simulink model "wrench_observer"  (R2018b)
settings: Solver=VariableStepAuto  StartTime=0.0  StopTime=0.75  RelTol=1e-3
InitFcn:
  | %x_k1 = 0.00001*ones(36,1); % initialisation with initial state uncertainity
  | %P_k1 = 0.00001*ones(36); % initialisation with initial state uncertainity
values from neighbouring files (symbols this model uses):
  a_noise = 0    [parameter.m]
  alpha1 = pi/2    (= 1.57079632679)    [parameter.m]
  alpha2 = 0    [parameter.m]
  alpha3 = 0    [parameter.m]
  angular_noise = 0    [parameter.m]
  g = 9.81    [parameter.m]
  K_f_comm = 1    [parameter.m]
  K_I = [500*eye(3), zeros(3), zeros(3) ... (first row only)    [parameter.m]
  K_tau_comm = 1    [parameter.m]
  K_tau_man_comm = 1    [parameter.m]
  m = 3.9    [parameter.m]
  m_l1 = 0.3    [parameter.m]
  m_l2 = 0.35    [parameter.m]
  m_l3 = 0.35    [parameter.m]
  N_m = 1*diag([(p_noise/(3*noise_factor))^2 (p_noise/(3*noise_factor))^2 (p_noise/(3*noise_factor))^2 (a_noise/(3*noise_factor))^2 (a_noise/(3*noise_factor))^2 (a_noise/(3*noise_factor))^2 (angular_noise/(3*noise_factor))^2 (angular_noise/(3*noise_factor))^2 (angular_noise/(3*noise_factor))^2 (omega_noise/(3*noise_factor))^2 (omega_noise/(3*noise_factor))^2 (omega_noise/(3*noise_factor))^2 (theta_noise/( ...(+272 chars)    [parameter.m]
  N_p = diag(noise_factor_EKF)    [parameter.m]
  omega_dot_noise = 0    [parameter.m]
  omega_noise = 0    [parameter.m]
  p_L1_l1 = [p_L1_x_l1 p_L1_y_l1 p_L1_z_l1]'    [parameter.m]
  p_L2_l2 = [p_L2_x_l2 p_L2_y_l2 p_L2_z_l2]'    [parameter.m]
  p_L3_l3 = [p_L3_x_l3 p_L3_y_l3 p_L3_z_l3]'    [parameter.m]
  p_noise = 0    [parameter.m]
  R_B_L0 = [1 0 0;0 1 0; 0 0 1]    [parameter.m]
  T_delay = 0    [parameter.m]
  T_dis = 0.01    [parameter.m]
  theta_dot_dot_noise = 0    [parameter.m]
  theta_dot_noise = 0    [parameter.m]
  theta_noise = 0    [parameter.m]
  Ts = 1/250    (= 0.004)    [parameter.m]
  v_noise = 0    [parameter.m]
libraries: simulink x9, dspstat3 x2, dspinverses x1
(part 5 of 5)

== matlab function wrench_observer/Motion Equations with Manipulator /MATLAB Function2 ==
  data: q input; G output; alpha1 parameter; alpha2 parameter; alpha3 parameter; R_B_L0 parameter; g parameter; m parameter; m_l2 parameter; m_l3 parameter; m_l1 parameter; p_L1_l1 parameter; p_L2_l2 parameter; p_L3_l3 parameter
function G = Gravity_Matrix(q, alpha1, alpha2, alpha3, R_B_L0, g, m, m_l2, m_l3, m_l1, p_L1_l1, p_L2_l2, p_L3_l3)
phi_E = q(4);
theta_E = q(5);
psi_E = q(6);
theta1 = q(7);
theta2 = q(8);
theta3 = q(9);
% theta4 = q(10);
% theta5 = q(11);

sphi = sin(phi_E); cphi = cos(phi_E);
sth = sin(theta_E); cth = cos(theta_E);
spsi = sin(psi_E); cpsi = cos(psi_E);
sth1 = sin(theta1); cth1 = cos(theta1); sth2 = sin(theta2); cth2 = cos(theta2); sth3 = sin(theta3); cth3 = cos(theta3);
salp1 = sin(alpha1); calp1 = cos(alpha1); salp2 = sin(alpha2); calp2 = cos(alpha2); salp3 = sin(alpha3); calp3 = cos(alpha3);

p_L1_x_l1 = p_L1_l1(1); p_L1_y_l1 = p_L1_l1(2); p_L1_z_l1 = p_L1_l1(3);
p_L2_x_l2 = p_L2_l2(1); p_L2_y_l2 = p_L2_l2(2); p_L2_z_l2 = p_L2_l2(3);
p_L3_x_l3 = p_L3_l3(1); p_L3_y_l3 = p_L3_l3(2); p_L3_z_l3 = p_L3_l3(3);
%% Rotation matrix from inertial to body frame
R_IB = [cpsi*cth cpsi*sth*sphi-spsi*cphi cpsi*sth*cphi+spsi*sphi;
        spsi*cth spsi*sth*sphi+cpsi*cphi spsi*sth*cphi-cpsi*sphi;
        -sth cth*sphi cth*cphi];

%% Rotation matrices from link i to manipulator base {L0}
% R_th_1 = [cth1 -sth1 0 0;
%     sth1 cth1 0 0;
%     0 0 1 0;
%     0 0 0 1];
% R_alpha_1 = [1 0 0 0;
%     0 calp1 -salp1 0;
%     0 salp1 calp1 0;
%     0 0 0 1];
% R_th_2 = [cth2 -sth2 0 0;
%     sth2 cth2 0 0;
%     0 0 1 0;
%     0 0 0 1];
% R_alpha_2 = [1 0 0 0;
%     0 calp2 -salp2 0;
%     0 salp2 calp2 0;
%     0 0 0 1];
% R_th_3 = [cth3 -sth3 0 0;
%     sth3 cth3 0 0;
%     0 0 1 0;
%     0 0 0 1];
% R_alpha_3 = [1 0 0 0;
%     0 calp3 -salp3 0;
%     0 salp3 calp3 0;
%     0 0 0 1];
% R_th_4 = [cth4 -sth4 0 0;
%         sth4 cth4 0 0;
%         0 0 1 0;
%         0 0 0 1];
% R_alpha_4 = [1 0 0 0;
%            0 calph4 -salph4 0;
%            0 salph4 calph4 0;
%            0 0 0 1];
% R_th_5 = [cth5 -sth5 0 0;
%         sth5 cth5 0 0;
%         0 0 1 0;
%         0 0 0 1];
% R_alpha_5 = [1 0 0 0;
%            0 calph5 -salph5 0;
%            0 salph5 calph5 0;
%            0 0 0 1];

% transformation matrices from link i to link i-1
% T_L0_L1 = R_th_1 * [1 0 0 0;0 1 0 0;0 0 1 d1;0 0 0 0] * [1 0 0 a1;0 1 0 0;0 0 1 0;0 0 0 1] * R_alpha_1;
% T_L1_L2 = R_th_2 * [1 0 0 0;0 1 0 0;0 0 1 d2;0 0 0 0] * [1 0 0 a2;0 1 0 0;0 0 1 0;0 0 0 1] * R_alpha_2;
% T_L2_L3 = R_th_3 * [1 0 0 0;0 1 0 0;0 0 1 d3;0 0 0 0] * [1 0 0 a3;0 1 0 0;0 0 1 0;0 0 0 1] * R_alpha_3;
% T_L3_L4 = R_th_4 * [1 0 0 0;0 1 0 0;0 0 1 d4;0 0 0 0] * [1 0 0 a4;0 1 0 0;0 0 1 0;0 0 0 1] * R_alpha_4;
% T_L4_L5 = R_th_5 * [1 0 0 0;0 1 0 0;0 0 1 d5;0 0 0 0] * [1 0 0 a5;0 1 0 0;0 0 1 0;0 0 0 1] * R_alpha_5;

% transformatin matrices from link i to manipulator base {L0}
% T_L0_L2 = T_L0_L1*T_L1_L2;
% T_L0_L3 = T_L0_L2*T_L2_L3;
% T_L0_L4 = T_L0_L3*T_L3_L4;
% T_L0_L5 = T_L0_L4*T_L4_L5;

% rotation matrices from link i to manipulator base {L0}
% R_L0_L1 = T_L0_L1(1:3,1:3);
% R_L0_L2 = T_L0_L2(1:3,1:3);
% R_L0_L3 = T_L0_L3(1:3,1:3);
% R_L0_L4 = T_L0_L4(1:3,1:3);
% R_L0_L5 = T_L0_L5(1:3,1:3);

R_L0_L1 = [ cth1, -calp1*sth1,  sth1*salp1;
            sth1,  cth1*calp1, -cth1*salp1;
             0,         salp1,       calp1];

R_L0_L2 = [ cth1*cth2 - calp1*sth1*sth2, sth1*salp1*salp2 - cth1*calp2*sth2 - cth2*calp1*calp2*sth1, cth1*sth2*salp2 + calp2*sth1*salp1 + cth2*calp1*sth1*salp2;
            cth2*sth1 + cth1*calp1*sth2, cth1*cth2*calp1*calp2 - cth1*salp1*salp2 - calp2*sth1*sth2, sth1*sth2*salp2 - cth1*calp2*salp1 - cth1*cth2*calp1*salp2;
             sth2*salp1,                                                   calp1*salp2 + cth2*calp2*salp1,                       calp1*calp2 - cth2*salp1*salp2];
         
R_L0_L3 = [ cth3*(cth1*cth2 - calp1*sth1*sth2) - sth3*(calp2*cth1*sth2 - salp1*salp2*sth1 + calp1*calp2*cth2*sth1),   salp3*(calp2*salp1*sth1 + salp2*cth1*sth2 + calp1*salp2*cth2*sth1) - calp3*cth3*(calp2*cth1*sth2 - salp1*salp2*sth1 + calp1*calp2*cth2*sth1) - calp3*sth3*(cth1*cth2 - calp1*sth1*sth2), calp3*(calp2*salp1*sth1 + salp2*cth1*sth2 + calp1*salp2*cth2*sth1) + salp3*cth3*(calp2*cth1*sth2 - salp1*salp2*sth1 + calp1*calp2*cth2*sth1) + salp3*sth3*(cth1*cth2 - calp1*sth1*sth2);
            cth3*(cth2*sth1 + calp1*cth1*sth2) - sth3*(salp1*salp2*cth1 + calp2*sth1*sth2 - calp1*calp2*cth1*cth2), - salp3*(calp2*salp1*cth1 - salp2*sth1*sth2 + calp1*salp2*cth1*cth2) - calp3*cth3*(salp1*salp2*cth1 + calp2*sth1*sth2 - calp1*calp2*cth1*cth2) - calp3*sth3*(cth2*sth1 + calp1*cth1*sth2), salp3*cth3*(salp1*salp2*cth1 + calp2*sth1*sth2 - calp1*calp2*cth1*cth2) - calp3*(calp2*salp1*cth1 - salp2*sth1*sth2 + calp1*salp2*cth1*cth2) + salp3*sth3*(cth2*sth1 + calp1*cth1*sth2);
             sth3*(calp1*salp2 + calp2*salp1*cth2) + salp1*cth3*sth2,                                                                                                                                      salp3*(calp1*calp2 - salp1*salp2*cth2) + calp3*cth3*(calp1*salp2 + calp2*salp1*cth2) - calp3*salp1*sth2*sth3,                                                                 calp3*(calp1*calp2 - salp1*salp2*cth2) - salp3*cth3*(calp1*salp2 + calp2*salp1*cth2) + salp1*salp3*sth2*sth3];

%% Gravity vector
a = R_B_L0(1,1)*R_IB(3,1)+ R_B_L0(2,1)*R_IB(3,2)+ R_B_L0(3,1)*R_IB(3,3);
b = R_B_L0(1,2)*R_IB(3,1)+ R_B_L0(2,2)*R_IB(3,2)+ R_B_L0(3,2)*R_IB(3,3);
c = R_B_L0(1,3)*R_IB(3,1)+ R_B_L0(2,3)*R_IB(3,2)+ R_B_L0(3,3)*R_IB(3,3);
% partial derivatives
dadphi = -R_B_L0(2,1)*cphi*cth + R_B_L0(3,1)*sphi*cth;
dadth = R_B_L0(1,1)*cth + R_B_L0(2,1)*sphi*sth + R_B_L0(3,1)*cphi*sth;
dadpsi = 0;
dbdphi = -R_B_L0(2,2)*cphi*cth + R_B_L0(3,2)*sphi*cth;
dbdth = R_B_L0(1,2)*cth + R_B_L0(2,2)*sphi*sth + R_B_L0(3,2)*cphi*sth;
dbdpsi = 0;
dcdphi = -R_B_L0(2,3)*cphi*cth + R_B_L0(3,3)*sphi*cth;
dcdth = R_B_L0(1,3)*cth + R_B_L0(2,3)*sphi*sth + R_B_L0(3,3)*cphi*sth;
dcdpsi = 0;

% gravity vector UAV
dUuav = [0 0 g*m 0 0 0 0 0 0]';
% gravity vector link 1
dUman_1 = zeros(9,1);
dUman_1(1) = 0; dUman_1(2) = 0; dUman_1(3) = g*m_l1;
dUman_1(4) = p_L1_x_l1*m_l1*g*(R_L0_L1(1,1)*dadphi + R_L0_L1(2,1)*dbdphi + R_L0_L1(3,1)*dcdphi)                                       + p_L1_y_l1*m_l1*g*(R_L0_L1(1,2)*dadphi + R_L0_L1(2,2)*dbdphi + R_L0_L1(3,2)*dcdphi)      + p_L1_z_l1*m_l1*g*(R_L0_L1(1,3)*dadphi + R_L0_L1(2,3)*dbdphi + R_L0_L1(3,3)*dcdphi);
dUman_1(5) = p_L1_x_l1*m_l1*g*(R_L0_L1(1,1)*dadth + R_L0_L1(2,1)*dbdth + R_L0_L1(3,1)*dcdth)                                          + p_L1_y_l1*m_l1*g*(R_L0_L1(1,2)*dadth + R_L0_L1(2,2)*dbdth + R_L0_L1(3,2)*dcdth)         + p_L1_z_l1*m_l1*g*(R_L0_L1(1,3)*dadth + R_L0_L1(2,3)*dbdth + R_L0_L1(3,3)*dcdth);
dUman_1(6) = p_L1_x_l1*m_l1*g*(R_L0_L1(1,1)*dadpsi + R_L0_L1(2,1)*dbdpsi + R_L0_L1(3,1)*dcdpsi)                                       + p_L1_y_l1*m_l1*g*(R_L0_L1(1,2)*dadpsi + R_L0_L1(2,2)*dbdpsi + R_L0_L1(3,2)*dcdpsi)      + p_L1_z_l1*m_l1*g*(R_L0_L1(1,3)*dadpsi + R_L0_L1(2,3)*dbdpsi + R_L0_L1(3,3)*dcdpsi);
dUman_1(7) = p_L1_x_l1*m_l1*g*(sth1*a - cth1*b)                                                                                       + p_L1_y_l1*m_l1*g*(-cth1*calp1*a + sth1*calp1*b)                                         + p_L1_z_l1*m_l1*g*(cth1*salp1*a + sth1*salp1*b);
dUman_1(8) = 0;
dUman_1(9) = 0;
% gravity vector link 2
dUman_2 = zeros(9,1);
dUman_2(1) = 0; dUman_2(2) = 0; dUman_2(3) = g*m_l2;
dUman_2(4) = p_L2_x_l2*m_l2*g*(R_L0_L2(1,1)*dadphi + R_L0_L2(2,1)*dbdphi + R_L0_L2(3,1)*dcdphi)                                       + p_L2_y_l2*m_l2*g*(R_L0_L2(1,2)*dadphi + R_L0_L2(2,2)*dbdphi + R_L0_L2(3,2)*dcdphi)                                                                  + p_L2_z_l2*m_l2*g*(R_L0_L2(1,3)*dadphi + R_L0_L2(2,3)*dbdphi + R_L0_L2(3,3)*dcdphi);
dUman_2(5) = p_L2_x_l2*m_l2*g*(R_L0_L2(1,1)*dadth + R_L0_L2(2,1)*dbdth + R_L0_L2(3,1)*dcdth)                                          + p_L2_y_l2*m_l2*g*(R_L0_L2(1,2)*dadth + R_L0_L2(2,2)*dbdth + R_L0_L2(3,2)*dcdth)                                                                     + p_L2_z_l2*m_l2*g*(R_L0_L2(1,3)*dadth + R_L0_L2(2,3)*dbdth + R_L0_L2(3,3)*dcdth);
dUman_2(6) = p_L2_x_l2*m_l2*g*(R_L0_L2(1,1)*dadpsi + R_L0_L2(2,1)*dbdpsi + R_L0_L2(3,1)*dcdpsi)                                       + p_L2_y_l2*m_l2*g*(R_L0_L2(1,2)*dadpsi + R_L0_L2(2,2)*dbdpsi + R_L0_L2(3,2)*dcdpsi)                                                                  + p_L2_z_l2*m_l2*g*(R_L0_L2(1,3)*dadpsi + R_L0_L2(2,3)*dbdpsi + R_L0_L2(3,3)*dcdpsi);
dUman_2(7) = p_L2_x_l2*m_l2*g*((sth1*cth2+cth1*sth2*calp1)*a + (-cth1*cth2+sth1*sth2*calp1)*b)                                        + p_L2_y_l2*m_l2*g*((-cth1*salp1*salp2-sth1*sth2*calp2+cth1*cth2*calp1*calp2)*a + (sth1*cth2*calp1*calp2-sth1*salp1*salp2+cth1*sth2*calp2)*b)         + p_L2_z_l2*m_l2*g*((sth1*sth2*salp2-cth2*salp1*calp2-cth1*cth2*calp1*salp2)*a + (-cth1*sth2*salp2-sth1*salp1*calp2-sth1*cth2*calp1*salp2)*b);
dUman_2(8) = p_L2_x_l2*m_l2*g*((sth2*cth1+cth2*sth1*calp1)*a + (sth2*sth1-cth2*cth1*calp1)*b + (-cth2*salp1)*c)                       + p_L2_y_l2*m_l2*g*((cth2*cth1*calp2-sth2*sth1*calp1*calp2)*a + (sth2*cth1*calp1*calp2+cth2*sth1*calp2)*b + (sth2*salp1*calp2)*c)                     + p_L2_z_l2*m_l2*g*((-cth2*cth1*salp2+sth2*sth1*calp1*salp2)*a + (-cth2*sth1*salp2)*b + (-sth2*salp1*salp2)*c);
dUman_2(9) = 0;
% gravity vector link 3
dUman_3 = zeros(9,1);
dUman_3(1) = 0; dUman_3(2) = 0; dUman_3(3) = g*m_l3;
dUman_3(4) = p_L3_x_l3*m_l3*g*(R_L0_L3(1,1)*dadphi + R_L0_L3(2,1)*dbdphi + R_L0_L3(3,1)*dcdphi)                                                                                                                                                                                                         + p_L3_y_l3*m_l3*g*(R_L0_L3(1,2)*dadphi + R_L0_L3(2,2)*dbdphi + R_L0_L3(3,2)*dcdphi)                                                                                                                                                                                                                                                                                            + p_L3_z_l3*m_l3*g*(R_L0_L3(1,3)*dadphi + R_L0_L3(2,3)*dbdphi + R_L0_L3(3,3)*dcdphi);
dUman_3(5) = p_L3_x_l3*m_l3*g*(R_L0_L3(1,1)*dadth + R_L0_L3(2,1)*dbdth + R_L0_L3(3,1)*dcdth)                                                                                                                                                                                                            + p_L3_y_l3*m_l3*g*(R_L0_L3(1,2)*dadth + R_L0_L3(2,2)*dbdth + R_L0_L3(3,2)*dcdth)                                                                                                                                                                                                                                                                                               + p_L3_z_l3*m_l3*g*(R_L0_L3(1,3)*dadth + R_L0_L3(2,3)*dbdth + R_L0_L3(3,3)*dcdth);
dUman_3(6) = p_L3_x_l3*m_l3*g*(R_L0_L3(1,1)*dadpsi + R_L0_L3(2,1)*dbdpsi + R_L0_L3(3,1)*dcdpsi)                                                                                                                                                                                                         + p_L3_y_l3*m_l3*g*(R_L0_L3(1,2)*dadpsi + R_L0_L3(2,2)*dbdpsi + R_L0_L3(3,2)*dcdpsi)                                                                                                                                                                                                                                                                                            + p_L3_z_l3*m_l3*g*(R_L0_L3(1,3)*dadpsi + R_L0_L3(2,3)*dbdpsi + R_L0_L3(3,3)*dcdpsi);
dUman_3(7) = p_L3_x_l3*m_l3*g*((sth1*cth2*cth3+cth1*sth2*calp1-sth1*sth2*sth3*calp2+cth1*salp1*salp2-cth1*cth2*calp1*calp2)*a + (cth1*cth2*cth3+cth1*sth2*calp1+cth1*sth2*sth3*calp2-sth1*salp1*salp2-sth1*cth2*calp1*calp2)*b)                                                                         + p_L3_y_l3*m_l3*g*((sth1*sth2*salp2*salp3-cth1*salp1*calp2-cth1*cth2*calp1*calp2-sth1*sth2*cth3*calp2*calp3+cth1*salp1*salp2-cth1*cth2*calp1*calp2-sth1*cth2*sth3*calp3+cth1*sth2*calp1)*a + (-sth1*salp1*calp2*salp3+cth1*sth2*salp2+sth1*cth2*calp1*salp2+cth1*sth2*cth3*calp2*calp3+sth1*salp1*salp2-sth1*cth2*calp1*calp2+cth1*cth2*sth3*calp3+sth1*sth2*calp1)*b)         + p_L3_z_l3*m_l3*g*((sth1*sth2*salp2*calp3-cth1*salp1*calp2-cth1*cth2*calp1*salp2+sth1*sth2*cth3*calp2*salp3+cth1*salp1*salp2-cth1*cth2*calp1*calp2+sth1*cth2*sth3*salp3+cth1*sth2*calp1)*a + (-cth1*sth2*cth3*calp2*salp3+sth1*salp1*salp2-sth1*cth2*calp1*calp2-sth1*salp1*calp2*calp3+cth1*sth2*salp2+sth1*cth2*calp1*salp2-cth1*cth2*sth3*salp3+sth1*sth2*calp1)*b);
dUman_3(8) = p_L3_x_l3*m_l3*g*((sth2*cth1*cth3+cth2*sth1*calp1+cth2*cth1*sth3*calp2+sth2*sth1*calp1)*a + (sth2*sth1*cth3-cth2*cth1*calp1+cth2*sth1*sth3*calp2-sth2*cth1*calp1*calp2)*b + (-cth2*cth3*salp1+sth2*sth3*salp1*calp2)*c)                                                                    + p_L3_y_l3*m_l3*g*((-cth2*cth1*salp2*salp3+sth2*sth1*calp1-sth2*cth1*sth3*calp3+cth2*sth1*calp1+cth2*cth1*cth3*calp2*calp3+sth2*sth1*calp1)*a + (-cth2*sth1*salp2*salp3-sth2*cth1*calp1-sth2*sth1*sth3*calp3-cth2*cth1*calp1+cth2*sth1*cth3*calp2*calp3-sth2*cth1*calp1)*b + (sth2*cth3*salp1*calp2*calp3+cth2*sth3*salp1*calp3-sth2*salp1*salp2*salp3)*c)                     + p_L3_z_l3*m_l3*g*((sth2*cth1*sth3*salp3+cth2*sth1*calp1-cth2*cth1*salp2*calp3+sth2*sth1*calp1-cth2*cth1*cth3*calp2*salp3+sth2*sth1*calp1)*a - (sth2*sth1*sth3*salp3-cth2*cth1*calp1-cth2*sth1*salp2*calp3-sth2*cth1*calp1-cth2*sth1*cth3*calp2*salp3-sth2*cth1*calp1)*b + (-cth2*sth3*salp1*salp3-sth2*salp1*salp2*calp3-sth2*cth3*salp1*calp2*salp3)*c);
dUman_3(9) = p_L3_x_l3*m_l3*g*((sth3*(cth1*cth2-sth1*sth2*calp1)+cth3*(cth1*sth2*calp2-sth1*salp1*salp2+sth1*cth2*calp1*calp2))*a + (sth3*(sth1*cth2+cth1*sth2*calp1)+cth3*(cth1*salp1*salp2+sth1*sth2*calp2-cth1*cth2*calp1*calp2))*b + (-cth3*(calp1*salp2+cth2*salp1*calp2)+sth3*sth2*salp1)*c)      + p_L3_y_l3*m_l3*g*((-sth3*calp3*(cth1*sth2*calp2-sth1*salp1*salp2+sth1*cth2*calp1*calp2-calp3*(cth1*cth2-sth1*sth2*calp1))*a + (-sth3*calp3*(cth1*salp1*salp2+sth1*sth2*calp2-cth1*cth2*calp1*calp2+cth3*calp3*(sth1*cth2+cth1*sth2*calp1)))*b + (-sth3*calp3*(calp1*salp2+cth2*salp1*calp2)+cth3*sth2*salp1*calp3))*c)                                                        + p_L3_z_l3*m_l3*g*((sth3*salp3*(cth1*sth2*calp2-sth1*salp1*salp2+sth1*cth2*calp1*calp2)-cth3*salp3*(cth1*cth2-sth1*sth2*calp1)))*a +(sth3*salp3*(cth1*salp1*salp2+sth1*sth2*calp2-cth1*cth2+calp1*calp2)-cth3*salp3*(sth1*cth2+cth1*sth2*calp1))*b + (-cth3*sth2*salp1*salp3-sth3*salp3*(calp1*salp2+cth2*salp1*calp2)*c);

G = dUuav + dUman_1 + dUman_2 + dUman_3;

== matlab function wrench_observer/Wrench Observer Hybrid Observer/Coriolis_Matrix/Coriolis_Matrix_simplified/MATLAB Function ==
  data: C11 input; C output; C12 input; C13 input; C21 input; C22 input; C23 input; C31 input; C32 input; C33 input
function C = Coriolis_Matrix(C11,C12,C13,C21,C22,C23,C31,C32,C33)
C = zeros(9);
C = [C11,C12,C13;C21,C22,C23;C31,C32,C33];

== matlab function wrench_observer/Wrench Observer Hybrid Observer/MATLAB Function2 ==
  data: q_meas input; G_est output; alpha1 parameter; alpha2 parameter; alpha3 parameter; R_B_L0 parameter; g parameter; m parameter; m_l2 parameter; m_l3 parameter; m_l1 parameter; p_L1_l1 parameter; p_L2_l2 parameter; p_L3_l3 parameter
function G_est = Gravity_Matrix(q_meas, alpha1, alpha2, alpha3, R_B_L0, g, m, m_l2, m_l3, m_l1, p_L1_l1, p_L2_l2, p_L3_l3)
phi_E = q_meas(4);
theta_E = q_meas(5);
psi_E = q_meas(6);
theta1 = q_meas(7);
theta2 = q_meas(8);
theta3 = q_meas(9);
% theta4 = q(10);
% theta5 = q(11);

sphi = sin(phi_E); cphi = cos(phi_E);
sth = sin(theta_E); cth = cos(theta_E);
spsi = sin(psi_E); cpsi = cos(psi_E);
sth1 = sin(theta1); cth1 = cos(theta1); sth2 = sin(theta2); cth2 = cos(theta2); sth3 = sin(theta3); cth3 = cos(theta3);
salp1 = sin(alpha1); calp1 = cos(alpha1); salp2 = sin(alpha2); calp2 = cos(alpha2); salp3 = sin(alpha3); calp3 = cos(alpha3);

p_L1_x_l1 = p_L1_l1(1); p_L1_y_l1 = p_L1_l1(2); p_L1_z_l1 = p_L1_l1(3);
p_L2_x_l2 = p_L2_l2(1); p_L2_y_l2 = p_L2_l2(2); p_L2_z_l2 = p_L2_l2(3);
p_L3_x_l3 = p_L3_l3(1); p_L3_y_l3 = p_L3_l3(2); p_L3_z_l3 = p_L3_l3(3);
%% Rotation matrix from inertial to body frame
R_IB = [cpsi*cth cpsi*sth*sphi-spsi*cphi cpsi*sth*cphi+spsi*sphi;
        spsi*cth spsi*sth*sphi+cpsi*cphi spsi*sth*cphi-cpsi*sphi;
        -sth cth*sphi cth*cphi];

%% Rotation matrices from link i to manipulator base {L0}
% R_th_1 = [cth1 -sth1 0 0;
%     sth1 cth1 0 0;
%     0 0 1 0;
%     0 0 0 1];
% R_alpha_1 = [1 0 0 0;
%     0 calp1 -salp1 0;
%     0 salp1 calp1 0;
%     0 0 0 1];
% R_th_2 = [cth2 -sth2 0 0;
%     sth2 cth2 0 0;
%     0 0 1 0;
%     0 0 0 1];
% R_alpha_2 = [1 0 0 0;
%     0 calp2 -salp2 0;
%     0 salp2 calp2 0;
%     0 0 0 1];
% R_th_3 = [cth3 -sth3 0 0;
%     sth3 cth3 0 0;
%     0 0 1 0;
%     0 0 0 1];
% R_alpha_3 = [1 0 0 0;
%     0 calp3 -salp3 0;
%     0 salp3 calp3 0;
%     0 0 0 1];
% R_th_4 = [cth4 -sth4 0 0;
%         sth4 cth4 0 0;
%         0 0 1 0;
%         0 0 0 1];
% R_alpha_4 = [1 0 0 0;
%            0 calph4 -salph4 0;
%            0 salph4 calph4 0;
%            0 0 0 1];
% R_th_5 = [cth5 -sth5 0 0;
%         sth5 cth5 0 0;
%         0 0 1 0;
%         0 0 0 1];
% R_alpha_5 = [1 0 0 0;
%            0 calph5 -salph5 0;
%            0 salph5 calph5 0;
%            0 0 0 1];

% transformation matrices from link i to link i-1
% T_L0_L1 = R_th_1 * [1 0 0 0;0 1 0 0;0 0 1 d1;0 0 0 0] * [1 0 0 a1;0 1 0 0;0 0 1 0;0 0 0 1] * R_alpha_1;
% T_L1_L2 = R_th_2 * [1 0 0 0;0 1 0 0;0 0 1 d2;0 0 0 0] * [1 0 0 a2;0 1 0 0;0 0 1 0;0 0 0 1] * R_alpha_2;
% T_L2_L3 = R_th_3 * [1 0 0 0;0 1 0 0;0 0 1 d3;0 0 0 0] * [1 0 0 a3;0 1 0 0;0 0 1 0;0 0 0 1] * R_alpha_3;
% T_L3_L4 = R_th_4 * [1 0 0 0;0 1 0 0;0 0 1 d4;0 0 0 0] * [1 0 0 a4;0 1 0 0;0 0 1 0;0 0 0 1] * R_alpha_4;
% T_L4_L5 = R_th_5 * [1 0 0 0;0 1 0 0;0 0 1 d5;0 0 0 0] * [1 0 0 a5;0 1 0 0;0 0 1 0;0 0 0 1] * R_alpha_5;

% transformatin matrices from link i to manipulator base {L0}
% T_L0_L2 = T_L0_L1*T_L1_L2;
% T_L0_L3 = T_L0_L2*T_L2_L3;
% T_L0_L4 = T_L0_L3*T_L3_L4;
% T_L0_L5 = T_L0_L4*T_L4_L5;

% rotation matrices from link i to manipulator base {L0}
% R_L0_L1 = T_L0_L1(1:3,1:3);
% R_L0_L2 = T_L0_L2(1:3,1:3);
% R_L0_L3 = T_L0_L3(1:3,1:3);
% R_L0_L4 = T_L0_L4(1:3,1:3);
% R_L0_L5 = T_L0_L5(1:3,1:3);

R_L0_L1 = [ cth1, -calp1*sth1,  sth1*salp1;
            sth1,  cth1*calp1, -cth1*salp1;
             0,         salp1,       calp1];

R_L0_L2 = [ cth1*cth2 - calp1*sth1*sth2, sth1*salp1*salp2 - cth1*calp2*sth2 - cth2*calp1*calp2*sth1, cth1*sth2*salp2 + calp2*sth1*salp1 + cth2*calp1*sth1*salp2;
            cth2*sth1 + cth1*calp1*sth2, cth1*cth2*calp1*calp2 - cth1*salp1*salp2 - calp2*sth1*sth2, sth1*sth2*salp2 - cth1*calp2*salp1 - cth1*cth2*calp1*salp2;
             sth2*salp1,                                                   calp1*salp2 + cth2*calp2*salp1,                       calp1*calp2 - cth2*salp1*salp2];
         
R_L0_L3 = [ cth3*(cth1*cth2 - calp1*sth1*sth2) - sth3*(calp2*cth1*sth2 - salp1*salp2*sth1 + calp1*calp2*cth2*sth1),   salp3*(calp2*salp1*sth1 + salp2*cth1*sth2 + calp1*salp2*cth2*sth1) - calp3*cth3*(calp2*cth1*sth2 - salp1*salp2*sth1 + calp1*calp2*cth2*sth1) - calp3*sth3*(cth1*cth2 - calp1*sth1*sth2), calp3*(calp2*salp1*sth1 + salp2*cth1*sth2 + calp1*salp2*cth2*sth1) + salp3*cth3*(calp2*cth1*sth2 - salp1*salp2*sth1 + calp1*calp2*cth2*sth1) + salp3*sth3*(cth1*cth2 - calp1*sth1*sth2);
            cth3*(cth2*sth1 + calp1*cth1*sth2) - sth3*(salp1*salp2*cth1 + calp2*sth1*sth2 - calp1*calp2*cth1*cth2), - salp3*(calp2*salp1*cth1 - salp2*sth1*sth2 + calp1*salp2*cth1*cth2) - calp3*cth3*(salp1*salp2*cth1 + calp2*sth1*sth2 - calp1*calp2*cth1*cth2) - calp3*sth3*(cth2*sth1 + calp1*cth1*sth2), salp3*cth3*(salp1*salp2*cth1 + calp2*sth1*sth2 - calp1*calp2*cth1*cth2) - calp3*(calp2*salp1*cth1 - salp2*sth1*sth2 + calp1*salp2*cth1*cth2) + salp3*sth3*(cth2*sth1 + calp1*cth1*sth2);
             sth3*(calp1*salp2 + calp2*salp1*cth2) + salp1*cth3*sth2,                                                                                                                                      salp3*(calp1*calp2 - salp1*salp2*cth2) + calp3*cth3*(calp1*salp2 + calp2*salp1*cth2) - calp3*salp1*sth2*sth3,                                                                 calp3*(calp1*calp2 - salp1*salp2*cth2) - salp3*cth3*(calp1*salp2 + calp2*salp1*cth2) + salp1*salp3*sth2*sth3];

%% Gravity vector
a = R_B_L0(1,1)*R_IB(3,1)+ R_B_L0(2,1)*R_IB(3,2)+ R_B_L0(3,1)*R_IB(3,3);
b = R_B_L0(1,2)*R_IB(3,1)+ R_B_L0(2,2)*R_IB(3,2)+ R_B_L0(3,2)*R_IB(3,3);
c = R_B_L0(1,3)*R_IB(3,1)+ R_B_L0(2,3)*R_IB(3,2)+ R_B_L0(3,3)*R_IB(3,3);
% partial derivatives
dadphi = -R_B_L0(2,1)*cphi*cth + R_B_L0(3,1)*sphi*cth;
dadth = R_B_L0(1,1)*cth + R_B_L0(2,1)*sphi*sth + R_B_L0(3,1)*cphi*sth;
dadpsi = 0;
dbdphi = -R_B_L0(2,2)*cphi*cth + R_B_L0(3,2)*sphi*cth;
dbdth = R_B_L0(1,2)*cth + R_B_L0(2,2)*sphi*sth + R_B_L0(3,2)*cphi*sth;
dbdpsi = 0;
dcdphi = -R_B_L0(2,3)*cphi*cth + R_B_L0(3,3)*sphi*cth;
dcdth = R_B_L0(1,3)*cth + R_B_L0(2,3)*sphi*sth + R_B_L0(3,3)*cphi*sth;
dcdpsi = 0;

% gravity vector UAV
dUuav = [0 0 g*m 0 0 0 0 0 0]';
% gravity vector link 1
dUman_1 = zeros(9,1);
dUman_1(1) = 0; dUman_1(2) = 0; dUman_1(3) = g*m_l1;
dUman_1(4) = p_L1_x_l1*m_l1*g*(R_L0_L1(1,1)*dadphi + R_L0_L1(2,1)*dbdphi + R_L0_L1(3,1)*dcdphi)                                       + p_L1_y_l1*m_l1*g*(R_L0_L1(1,2)*dadphi + R_L0_L1(2,2)*dbdphi + R_L0_L1(3,2)*dcdphi)      + p_L1_z_l1*m_l1*g*(R_L0_L1(1,3)*dadphi + R_L0_L1(2,3)*dbdphi + R_L0_L1(3,3)*dcdphi);
dUman_1(5) = p_L1_x_l1*m_l1*g*(R_L0_L1(1,1)*dadth + R_L0_L1(2,1)*dbdth + R_L0_L1(3,1)*dcdth)                                          + p_L1_y_l1*m_l1*g*(R_L0_L1(1,2)*dadth + R_L0_L1(2,2)*dbdth + R_L0_L1(3,2)*dcdth)         + p_L1_z_l1*m_l1*g*(R_L0_L1(1,3)*dadth + R_L0_L1(2,3)*dbdth + R_L0_L1(3,3)*dcdth);
dUman_1(6) = p_L1_x_l1*m_l1*g*(R_L0_L1(1,1)*dadpsi + R_L0_L1(2,1)*dbdpsi + R_L0_L1(3,1)*dcdpsi)                                       + p_L1_y_l1*m_l1*g*(R_L0_L1(1,2)*dadpsi + R_L0_L1(2,2)*dbdpsi + R_L0_L1(3,2)*dcdpsi)      + p_L1_z_l1*m_l1*g*(R_L0_L1(1,3)*dadpsi + R_L0_L1(2,3)*dbdpsi + R_L0_L1(3,3)*dcdpsi);
dUman_1(7) = p_L1_x_l1*m_l1*g*(sth1*a - cth1*b)                                                                                       + p_L1_y_l1*m_l1*g*(-cth1*calp1*a + sth1*calp1*b)                                         + p_L1_z_l1*m_l1*g*(cth1*salp1*a + sth1*salp1*b);
dUman_1(8) = 0;
dUman_1(9) = 0;
% gravity vector link 2
dUman_2 = zeros(9,1);
dUman_2(1) = 0; dUman_2(2) = 0; dUman_2(3) = g*m_l2;
dUman_2(4) = p_L2_x_l2*m_l2*g*(R_L0_L2(1,1)*dadphi + R_L0_L2(2,1)*dbdphi + R_L0_L2(3,1)*dcdphi)                                       + p_L2_y_l2*m_l2*g*(R_L0_L2(1,2)*dadphi + R_L0_L2(2,2)*dbdphi + R_L0_L2(3,2)*dcdphi)                                                                  + p_L2_z_l2*m_l2*g*(R_L0_L2(1,3)*dadphi + R_L0_L2(2,3)*dbdphi + R_L0_L2(3,3)*dcdphi);
dUman_2(5) = p_L2_x_l2*m_l2*g*(R_L0_L2(1,1)*dadth + R_L0_L2(2,1)*dbdth + R_L0_L2(3,1)*dcdth)                                          + p_L2_y_l2*m_l2*g*(R_L0_L2(1,2)*dadth + R_L0_L2(2,2)*dbdth + R_L0_L2(3,2)*dcdth)                                                                     + p_L2_z_l2*m_l2*g*(R_L0_L2(1,3)*dadth + R_L0_L2(2,3)*dbdth + R_L0_L2(3,3)*dcdth);
dUman_2(6) = p_L2_x_l2*m_l2*g*(R_L0_L2(1,1)*dadpsi + R_L0_L2(2,1)*dbdpsi + R_L0_L2(3,1)*dcdpsi)                                       + p_L2_y_l2*m_l2*g*(R_L0_L2(1,2)*dadpsi + R_L0_L2(2,2)*dbdpsi + R_L0_L2(3,2)*dcdpsi)                                                                  + p_L2_z_l2*m_l2*g*(R_L0_L2(1,3)*dadpsi + R_L0_L2(2,3)*dbdpsi + R_L0_L2(3,3)*dcdpsi);
dUman_2(7) = p_L2_x_l2*m_l2*g*((sth1*cth2+cth1*sth2*calp1)*a + (-cth1*cth2+sth1*sth2*calp1)*b)                                        + p_L2_y_l2*m_l2*g*((-cth1*salp1*salp2-sth1*sth2*calp2+cth1*cth2*calp1*calp2)*a + (sth1*cth2*calp1*calp2-sth1*salp1*salp2+cth1*sth2*calp2)*b)         + p_L2_z_l2*m_l2*g*((sth1*sth2*salp2-cth2*salp1*calp2-cth1*cth2*calp1*salp2)*a + (-cth1*sth2*salp2-sth1*salp1*calp2-sth1*cth2*calp1*salp2)*b);
dUman_2(8) = p_L2_x_l2*m_l2*g*((sth2*cth1+cth2*sth1*calp1)*a + (sth2*sth1-cth2*cth1*calp1)*b + (-cth2*salp1)*c)                       + p_L2_y_l2*m_l2*g*((cth2*cth1*calp2-sth2*sth1*calp1*calp2)*a + (sth2*cth1*calp1*calp2+cth2*sth1*calp2)*b + (sth2*salp1*calp2)*c)                     + p_L2_z_l2*m_l2*g*((-cth2*cth1*salp2+sth2*sth1*calp1*salp2)*a + (-cth2*sth1*salp2)*b + (-sth2*salp1*salp2)*c);
dUman_2(9) = 0;
% gravity vector link 3
dUman_3 = zeros(9,1);
dUman_3(1) = 0; dUman_3(2) = 0; dUman_3(3) = g*m_l3;
dUman_3(4) = p_L3_x_l3*m_l3*g*(R_L0_L3(1,1)*dadphi + R_L0_L3(2,1)*dbdphi + R_L0_L3(3,1)*dcdphi)                                                                                                                                                                                                         + p_L3_y_l3*m_l3*g*(R_L0_L3(1,2)*dadphi + R_L0_L3(2,2)*dbdphi + R_L0_L3(3,2)*dcdphi)                                                                                                                                                                                                                                                                                            + p_L3_z_l3*m_l3*g*(R_L0_L3(1,3)*dadphi + R_L0_L3(2,3)*dbdphi + R_L0_L3(3,3)*dcdphi);
dUman_3(5) = p_L3_x_l3*m_l3*g*(R_L0_L3(1,1)*dadth + R_L0_L3(2,1)*dbdth + R_L0_L3(3,1)*dcdth)                                                                                                                                                                                                            + p_L3_y_l3*m_l3*g*(R_L0_L3(1,2)*dadth + R_L0_L3(2,2)*dbdth + R_L0_L3(3,2)*dcdth)                                                                                                                                                                                                                                                                                               + p_L3_z_l3*m_l3*g*(R_L0_L3(1,3)*dadth + R_L0_L3(2,3)*dbdth + R_L0_L3(3,3)*dcdth);
dUman_3(6) = p_L3_x_l3*m_l3*g*(R_L0_L3(1,1)*dadpsi + R_L0_L3(2,1)*dbdpsi + R_L0_L3(3,1)*dcdpsi)                                                                                                                                                                                                         + p_L3_y_l3*m_l3*g*(R_L0_L3(1,2)*dadpsi + R_L0_L3(2,2)*dbdpsi + R_L0_L3(3,2)*dcdpsi)                                                                                                                                                                                                                                                                                            + p_L3_z_l3*m_l3*g*(R_L0_L3(1,3)*dadpsi + R_L0_L3(2,3)*dbdpsi + R_L0_L3(3,3)*dcdpsi);
dUman_3(7) = p_L3_x_l3*m_l3*g*((sth1*cth2*cth3+cth1*sth2*calp1-sth1*sth2*sth3*calp2+cth1*salp1*salp2-cth1*cth2*calp1*calp2)*a + (cth1*cth2*cth3+cth1*sth2*calp1+cth1*sth2*sth3*calp2-sth1*salp1*salp2-sth1*cth2*calp1*calp2)*b)                                                                         + p_L3_y_l3*m_l3*g*((sth1*sth2*salp2*salp3-cth1*salp1*calp2-cth1*cth2*calp1*calp2-sth1*sth2*cth3*calp2*calp3+cth1*salp1*salp2-cth1*cth2*calp1*calp2-sth1*cth2*sth3*calp3+cth1*sth2*calp1)*a + (-sth1*salp1*calp2*salp3+cth1*sth2*salp2+sth1*cth2*calp1*salp2+cth1*sth2*cth3*calp2*calp3+sth1*salp1*salp2-sth1*cth2*calp1*calp2+cth1*cth2*sth3*calp3+sth1*sth2*calp1)*b)         + p_L3_z_l3*m_l3*g*((sth1*sth2*salp2*calp3-cth1*salp1*calp2-cth1*cth2*calp1*salp2+sth1*sth2*cth3*calp2*salp3+cth1*salp1*salp2-cth1*cth2*calp1*calp2+sth1*cth2*sth3*salp3+cth1*sth2*calp1)*a + (-cth1*sth2*cth3*calp2*salp3+sth1*salp1*salp2-sth1*cth2*calp1*calp2-sth1*salp1*calp2*calp3+cth1*sth2*salp2+sth1*cth2*calp1*salp2-cth1*cth2*sth3*salp3+sth1*sth2*calp1)*b);
dUman_3(8) = p_L3_x_l3*m_l3*g*((sth2*cth1*cth3+cth2*sth1*calp1+cth2*cth1*sth3*calp2+sth2*sth1*calp1)*a + (sth2*sth1*cth3-cth2*cth1*calp1+cth2*sth1*sth3*calp2-sth2*cth1*calp1*calp2)*b + (-cth2*cth3*salp1+sth2*sth3*salp1*calp2)*c)                                                                    + p_L3_y_l3*m_l3*g*((-cth2*cth1*salp2*salp3+sth2*sth1*calp1-sth2*cth1*sth3*calp3+cth2*sth1*calp1+cth2*cth1*cth3*calp2*calp3+sth2*sth1*calp1)*a + (-cth2*sth1*salp2*salp3-sth2*cth1*calp1-sth2*sth1*sth3*calp3-cth2*cth1*calp1+cth2*sth1*cth3*calp2*calp3-sth2*cth1*calp1)*b + (sth2*cth3*salp1*calp2*calp3+cth2*sth3*salp1*calp3-sth2*salp1*salp2*salp3)*c)                     + p_L3_z_l3*m_l3*g*((sth2*cth1*sth3*salp3+cth2*sth1*calp1-cth2*cth1*salp2*calp3+sth2*sth1*calp1-cth2*cth1*cth3*calp2*salp3+sth2*sth1*calp1)*a - (sth2*sth1*sth3*salp3-cth2*cth1*calp1-cth2*sth1*salp2*calp3-sth2*cth1*calp1-cth2*sth1*cth3*calp2*salp3-sth2*cth1*calp1)*b + (-cth2*sth3*salp1*salp3-sth2*salp1*salp2*calp3-sth2*cth3*salp1*calp2*salp3)*c);
dUman_3(9) = p_L3_x_l3*m_l3*g*((sth3*(cth1*cth2-sth1*sth2*calp1)+cth3*(cth1*sth2*calp2-sth1*salp1*salp2+sth1*cth2*calp1*calp2))*a + (sth3*(sth1*cth2+cth1*sth2*calp1)+cth3*(cth1*salp1*salp2+sth1*sth2*calp2-cth1*cth2*calp1*calp2))*b + (-cth3*(calp1*salp2+cth2*salp1*calp2)+sth3*sth2*salp1)*c)      + p_L3_y_l3*m_l3*g*((-sth3*calp3*(cth1*sth2*calp2-sth1*salp1*salp2+sth1*cth2*calp1*calp2-calp3*(cth1*cth2-sth1*sth2*calp1))*a + (-sth3*calp3*(cth1*salp1*salp2+sth1*sth2*calp2-cth1*cth2*calp1*calp2+cth3*calp3*(sth1*cth2+cth1*sth2*calp1)))*b + (-sth3*calp3*(calp1*salp2+cth2*salp1*calp2)+cth3*sth2*salp1*calp3))*c)                                                        + p_L3_z_l3*m_l3*g*((sth3*salp3*(cth1*sth2*calp2-sth1*salp1*salp2+sth1*cth2*calp1*calp2)-cth3*salp3*(cth1*cth2-sth1*sth2*calp1)))*a +(sth3*salp3*(cth1*salp1*salp2+sth1*sth2*calp2-cth1*cth2+calp1*calp2)-cth3*salp3*(sth1*cth2+cth1*sth2*calp1))*b + (-cth3*sth2*salp1*salp3-sth3*salp3*(calp1*salp2+cth2*salp1*calp2)*c);

G_est = dUuav + dUman_1 + dUman_2 + dUman_3;

== matlab function wrench_observer/Wrench Observer Hybrid Observer/MATLAB Function ==
  data: eul_angl input; m_12 output; theta input
function m_12 = m12(eul_angl,theta)
phi = eul_angl(1);
the = eul_angl(2);
psi = eul_angl(3);
theta1 = theta(1);
theta2 = theta(2);
theta3 = theta(3);
m_12 = [ 0,(phi^2*the*(3*sin(theta2 + theta3) + 3*sin(theta2) + 1))/40, -(3*phi^2*psi*the*sin(theta1)*(cos(theta2 + theta3) + cos(theta2)))/40;
-(phi*the*(3*sin(theta2 + theta3) + 3*sin(theta2) + 1))/40,0,(3*phi*psi*the^2*cos(theta1)*(cos(theta2 + theta3) + cos(theta2)))/40;
(3*phi*psi*sin(theta1)*(cos(theta2 + theta3) + cos(theta2)))/40, -(3*phi*psi*the*cos(theta1)*(cos(theta2 + theta3) + cos(theta2)))/40,0];

== matlab function wrench_observer/Wrench Observer Hybrid Observer/MATLAB Function1 ==
  data: eul_angl input; m_13 output; theta input
function m_13 = m13(eul_angl,theta)
phi = eul_angl(1);
the = eul_angl(2);
psi = eul_angl(3);
theta1 = theta(1);
theta2 = theta(2);
theta3 = theta(3);
m_13 = [-(3*psi*the*cos(theta1)*((3*sin(theta2 + theta3))/10 - 1/10))/2, -(3*psi*the*cos(theta1)*((3*sin(theta2 + theta3))/10 - (3*sin(theta2))/10))/2, 0;
 -(3*phi*psi*sin(theta1)*((3*sin(theta2 + theta3))/10 - 1/10))/2, -(3*phi*psi*sin(theta1)*((3*sin(theta2 + theta3))/10 - (3*sin(theta2))/10))/2, 0;
 (9*phi*the*cos(theta2 + theta3))/20,(3*phi*the*((3*cos(theta2 + theta3))/10 - (3*cos(theta2))/10))/2, 0];

== matlab function wrench_observer/Wrench Observer Hybrid Observer/MATLAB Function3 ==
  data: eul_angl input; c_12 output; theta input
function c_12 = c12(eul_angl,theta)
phi = eul_angl(1);
the = eul_angl(2);
psi = eul_angl(3);
theta1 = theta(1);
theta2 = theta(2);
theta3 = theta(3);
c_12 = [(3*phi^2*(psi + the)*(2*the + 7*cos(theta2)*sin(theta1) + 7*the*sin(theta2) - 7*sin(theta1)*sin(theta2)*sin(theta3) + 7*the*cos(theta2)*sin(theta3) + 7*the*cos(theta3)*sin(theta2) + 7*cos(theta2)*cos(theta3)*sin(theta1)))/800, (3*phi*(7*phi*the*cos(theta2) - 40*psi*the*cos(theta2) - 14*the*cos(theta1)*cos(theta2) + 7*phi*the*cos(theta2)*sin(theta1) - 14*phi*the*sin(theta2)*sin(theta3) - 80*psi*the*sin(theta2)*sin(theta3) - 14*the*cos(theta1)*cos(theta2)*cos(theta3) + 14*the*cos(theta1)*sin(theta2)*sin(theta3) + 14*phi*the*cos(theta2)*cos(theta3) + 80*psi*the*cos(theta2)*cos(theta3) + 7*phi*psi*cos(theta2)*sin(theta1) + 7*phi*psi*cos(theta2)*cos(theta3)*sin(theta1) + 7*phi*the*cos(theta2)*cos(theta3)*sin(theta1) - 7*phi*psi*sin(theta1)*sin(theta2)*sin(theta3) - 7*phi*the*sin(theta1)*sin(theta2)*sin(theta3)))/800, (phi*(12*phi*the^2 - 80*psi*sin(theta1) - 42*psi*the^2*cos(theta2 - theta1 + theta3) - 42*psi*the^2*cos(theta1 + theta2) + 42*phi*the^2*sin(theta2 + theta3) + 480*psi*sin(theta2 + theta3)*sin(theta1) + 42*phi*the^2*sin(theta2) - 240*psi*sin(theta1)*sin(theta2) - 42*psi*the^2*cos(theta1 - theta2) + 12*phi*psi*the - 42*psi*the^2*cos(theta1 + theta2 + theta3) + 21*phi*psi*the*cos(theta2 - theta1 + theta3) - 42*phi*psi*the*cos(theta1 + theta2) + 42*phi*psi*the*sin(theta2 + theta3) + 42*phi*psi*the*sin(theta2) - 63*phi*psi*the*cos(theta1 + theta2 + theta3)))/1600;
 (3*phi*psi*cos(theta2))/20 - (21*phi*the*cos(theta2))/800 + (21*the*cos(theta1)*cos(theta2))/800 - (21*phi*the*cos(theta2)*sin(theta1))/400 + (3*phi*psi*sin(theta2)*sin(theta3))/10 + (21*phi*the*sin(theta2)*sin(theta3))/400 + (21*the*cos(theta1)*cos(theta2)*cos(theta3))/800 - (21*the*cos(theta1)*sin(theta2)*sin(theta3))/800 - (3*phi*psi*cos(theta2)*cos(theta3))/10 - (21*phi*the*cos(theta2)*cos(theta3))/400 - (21*phi*psi*the*cos(theta1)*cos(theta2))/800 - (21*phi*the*cos(theta2)*cos(theta3)*sin(theta1))/400 + (21*phi*the*sin(theta1)*sin(theta2)*sin(theta3))/400 - (21*phi*psi*the*cos(theta1)*cos(theta2)*cos(theta3))/800 + (21*phi*psi*the*cos(theta1)*sin(theta2)*sin(theta3))/800, (3*the*(7*cos(theta1)*cos(theta2) + 2*phi*the + 7*cos(theta2 + theta3)*cos(theta1) + 2*phi^2*psi*the + 7*phi*the*sin(theta2) + 7*phi*the*sin(theta2 + theta3) - 7*phi*psi*cos(theta2 + theta3)*cos(theta1) + 7*phi^2*psi*the*sin(theta2 + theta3) - 7*phi*psi*cos(theta1)*cos(theta2) + 7*phi^2*psi*the*sin(theta2)))/800, (the*(12*phi*the + 80*psi*cos(theta1) + 12*phi^2*psi*the + 42*phi*the*sin(theta2) + 42*phi^2*psi*sin(theta2 - theta1 + theta3) - 42*phi^2*psi*sin(theta1 + theta2) - 480*psi*sin(theta2 + theta3)*cos(theta1) + 240*psi*cos(theta1)*sin(theta2) - 42*phi^2*psi*sin(theta1 - theta2) - 42*phi^2*psi*sin(theta1 + theta2 + theta3) + 42*phi*the*sin(theta2 + theta3) - 21*phi*psi*the*sin(theta2 - theta1 + theta3) - 42*phi*psi*the*sin(theta1 + theta2) + 42*phi^2*psi*the*sin(theta2 + theta3) - 63*phi*psi*the*sin(theta1 + theta2 + theta3) + 42*phi^2*psi*the*sin(theta2)))/1600;
 (phi*the*sin(theta1))/20 - (21*phi*psi*sin(theta2))/400 - (3*phi*psi)/200 + (21*psi*the*cos(theta1 - theta2))/1600 + (63*phi*psi*cos(theta1 + theta2 + theta3))/1600 + (21*psi*the*cos(theta1 + theta2 + theta3))/1600 - (21*phi*psi*cos(theta2 - theta1 + theta3))/1600 + (21*psi*the*cos(theta2 - theta1 + theta3))/1600 + (21*phi*psi*cos(theta1 + theta2))/800 + (21*psi*the*cos(theta1 + theta2))/1600 - (21*phi*psi*sin(theta2 + theta3))/400 + (3*phi*the*sin(theta1)*sin(theta2))/20 - (21*phi*psi*the^2*cos(theta1 - theta2))/1600 - (21*phi*psi*the^2*cos(theta1 + theta2 + theta3))/1600 - (21*phi*psi*the^2*cos(theta2 - theta1 + theta3))/1600 - (21*phi*psi*the^2*cos(theta1 + theta2))/1600 - (3*phi*the*sin(theta2 + theta3)*sin(theta1))/10, (the*cos(theta1)*((3*cos(theta2)*sin(theta3))/10 + (3*cos(theta3)*sin(theta2))/10 - 1/10))/2 - (3*phi^2*psi*the)/200 - (7*phi^2*psi*((3*sin(theta1)*sin(theta2)*sin(theta3))/20 - (3*cos(theta2)*cos(theta3)*sin(theta1))/20))/40 + (the*cos(theta1)*((3*cos(theta2)*sin(theta3))/10 - (3*sin(theta2))/10 + (3*cos(theta3)*sin(theta2))/10))/2 + (7*phi*psi*the*((3*cos(theta1)*cos(theta2)*sin(theta3))/20 + (3*cos(theta1)*cos(theta3)*sin(theta2))/20))/20 + (21*phi^2*psi*cos(theta2)*sin(theta1))/800 - (7*phi^2*psi*the*((3*cos(theta2)*sin(theta3))/20 + (3*cos(theta3)*sin(theta2))/20))/20 - (21*phi^2*psi*the*sin(theta2))/400 + (21*phi*psi*the*cos(theta1)*sin(theta2))/800,(21*psi*(cos(theta2 + theta3) + cos(theta2))*(sin(theta1)*phi^2 - cos(theta1)*phi*the^2 - sin(theta1)*phi*the + cos(theta1)*the))/800];

== matlab function wrench_observer/Wrench Observer Hybrid Observer/MATLAB Function4 ==
  data: eul_angl input; c_13 output; theta input
function c_13 = c13(eul_angl,theta)
phi = eul_angl(1);
the = eul_angl(2);
psi = eul_angl(3);
theta1 = theta(1);
theta2 = theta(2);
theta3 = theta(3);
c_13 = [ -(psi*(40*phi*sin(theta1) - 60*the*cos(theta2 - theta1 + theta3) - 60*the*cos(theta1 + theta2) - 60*phi*cos(theta2 - theta1 + theta3) + 80*the*sin(theta1) + 60*the*cos(theta1 - theta2) + 60*phi*cos(theta1 + theta2 + theta3) + 300*the*cos(theta1 + theta2 + theta3) + (21*phi^2*the*cos(theta2 - theta1 + theta3))/2 + (21*phi^2*the*cos(theta1 + theta2))/2 + (21*phi^2*the*cos(theta1 - theta2))/2 + (21*phi^2*the*cos(theta1 + theta2 + theta3))/2 - 120*phi*the*cos(theta2 + theta3)))/800, (21*phi^2*the*cos(theta2 + theta3))/800 + (21*phi^2*the*cos(theta2))/800 - psi*the*cos(theta1)*((3*cos(theta2 + theta3))/10 - (3*cos(theta2))/10) - (3*psi*the*cos(theta2 + theta3)*cos(theta1))/10 + (phi*psi*sin(theta1)*((3*sin(theta2 + theta3))/10 - (3*sin(theta2))/10))/2 + (psi*the*sin(theta1)*((3*sin(theta2 + theta3))/10 - (3*sin(theta2))/10))/2 + (3*phi*psi*the*(cos(theta2 + theta3) - cos(theta2)))/20 + (21*phi^2*psi*the*sin(theta2 + theta3)*sin(theta1))/800 + (21*phi^2*psi*the*sin(theta1)*sin(theta2))/800, (21*phi^2*the*cos(theta2 + theta3))/800 - (3*psi*the*cos(theta2 + theta3)*cos(theta1))/10 - (7*phi^2*psi*the*((3*cos(theta1 + theta2 + theta3))/40 - (3*cos(theta2 - theta1 + theta3))/40))/40;
-(psi*(60*the*sin(theta1 + theta2 + theta3) + 60*phi*sin(theta2 - theta1 + theta3) + 60*the*sin(theta2 - theta1 + theta3) + 120*phi*cos(theta2 + theta3) - 60*phi*sin(theta1 + theta2) - 80*phi*cos(theta1) - 40*the*cos(theta1) + 60*phi*sin(theta1 - theta2) + 300*phi*sin(theta1 + theta2 + theta3) - (21*phi*the^2*sin(theta2 - theta1 + theta3))/2 + (21*phi*the^2*sin(theta1 + theta2))/2 + (21*phi*the^2*sin(theta1 - theta2))/2 + (21*phi*the^2*sin(theta1 + theta2 + theta3))/2))/800, (3*phi*psi*cos(theta2))/20 - (21*phi*the*cos(theta2))/800 + (3*phi*psi*sin(theta1 - theta2))/40 - (3*psi*the*sin(theta1 - theta2))/40 - (3*phi*psi*sin(theta1 + theta2 + theta3))/8 - (3*psi*the*sin(theta1 + theta2 + theta3))/40 + (9*phi*psi*sin(theta2 - theta1 + theta3))/40 - (3*psi*the*sin(theta2 - theta1 + theta3))/40 - (3*phi*psi*cos(theta2 + theta3))/20 - (21*phi*the*cos(theta2 + theta3))/800 + (9*phi*psi*sin(theta1 + theta2))/40 + (3*psi*the*sin(theta1 + theta2))/40 + (21*phi*psi*the^2*sin(theta1 - theta2))/1600 - (21*phi*psi*the^2*sin(theta1 + theta2 + theta3))/1600 - (21*phi*psi*the^2*sin(theta2 - theta1 + theta3))/1600 - (21*phi*psi*the^2*sin(theta1 + theta2))/1600, - (21*phi*the*cos(theta2 + theta3))/800 - (3*phi*psi*cos(theta2 + theta3)*sin(theta1))/10 - (7*phi*psi*the^2*((3*sin(theta1 + theta2 + theta3))/40 + (3*sin(theta2 - theta1 + theta3))/40))/40;
(the*cos(theta1)*((3*sin(theta2 + theta3))/10 - 1/10))/2 - (3*phi*the*sin(theta2 + theta3))/10 - (phi*the*sin(theta1)*((3*sin(theta2 + theta3))/10 - 1/10))/2 + (21*phi*psi*cos(theta2 + theta3)*cos(theta1))/800 + (21*phi*psi*cos(theta1)*cos(theta2))/800 + (21*phi*psi*the*cos(theta2 + theta3)*sin(theta1))/800 + (21*phi*psi*the*cos(theta2)*sin(theta1))/800, (3*phi*the*sin(theta2))/10 - (3*the*cos(theta1)*sin(theta2))/20 - (3*phi*the*cos(theta2)*sin(theta3))/5 - (3*phi*the*cos(theta3)*sin(theta2))/5 - (21*phi*psi*sin(theta1)*sin(theta2))/800 + (3*phi*the*sin(theta1)*sin(theta2))/20 + (3*the*cos(theta1)*cos(theta2)*sin(theta3))/20 + (3*the*cos(theta1)*cos(theta3)*sin(theta2))/20 + (21*phi*psi*the*cos(theta1)*sin(theta2))/800 - (21*phi*psi*cos(theta2)*sin(theta1)*sin(theta3))/800 - (21*phi*psi*cos(theta3)*sin(theta1)*sin(theta2))/800 - (3*phi*the*cos(theta2)*sin(theta1)*sin(theta3))/20 - (3*phi*the*cos(theta3)*sin(theta1)*sin(theta2))/20 + (21*phi*psi*the*cos(theta1)*cos(theta2)*sin(theta3))/800 + (21*phi*psi*the*cos(theta1)*cos(theta3)*sin(theta2))/800, -(3*phi*sin(theta2 + theta3)*(80*the + 7*psi*sin(theta1) - 7*psi*the*cos(theta1)))/800];

== matlab function wrench_observer/Wrench Observer Mom. based Method/transpose ==
  data: C input; C_trans output
function C_trans = fcn(C)

C_trans = C';
